simulink library "GNC_math_lib"  (R2022b)
settings: Solver=VariableStepAuto  StartTime=0.0  StopTime=10.0  RelTol=1e-3
settings Model: Creator=David  LastModifiedBy=David

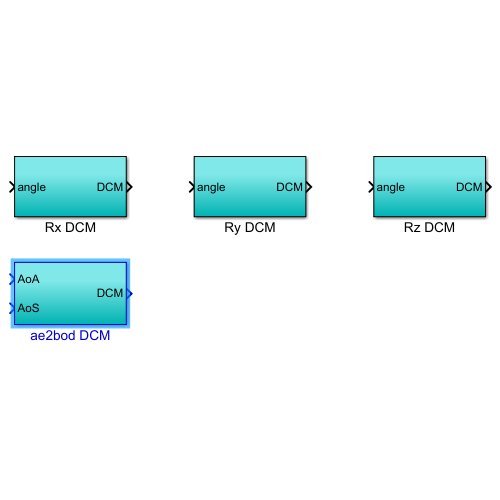
[thumbnail: Simulink's stored preview of the top-level diagram]
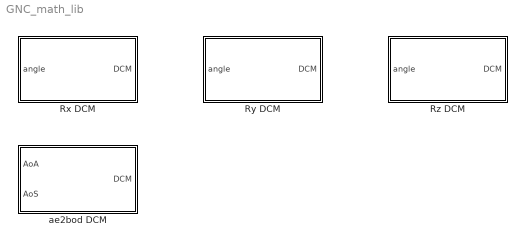
== system GNC_math_lib ==
  Rx DCM : Subsystem
  Ry DCM : Subsystem
  Rz DCM : Subsystem
  ae2bod DCM : Subsystem

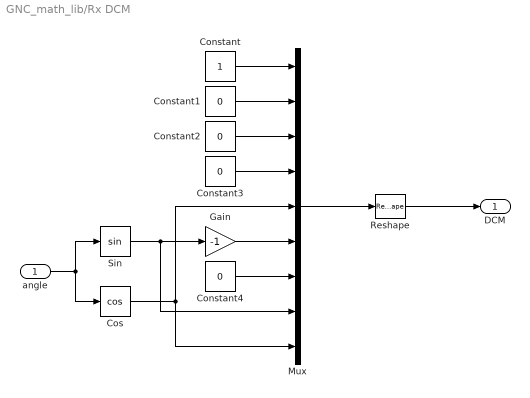
== system GNC_math_lib/Rx DCM ==
  angle : Inport
  Constant : Constant
  Constant{1..4} (4 alike) : Constant  Value=0
  Cos : Trigonometry  Operator=cos
  Gain : Gain  Gain=-1
  Mux : Mux  Inputs=9
  Reshape : Reshape  OutputDimensionality=Customize  OutputDimensions=[3,3]
  Sin : Trigonometry
  DCM : Outport
  wires:
  angle/1 -> Cos/1, Sin/1
  Reshape/1 -> DCM/1
  Mux/1 -> Reshape/1
  Constant/1 -> Mux/1
  Constant1/1 -> Mux/2
  Constant2/1 -> Mux/3
  Constant3/1 -> Mux/4
  Constant4/1 -> Mux/7
  Cos/1 -> Mux/9, Mux/5
  Sin/1 -> Mux/8, Gain/1
  Gain/1 -> Mux/6

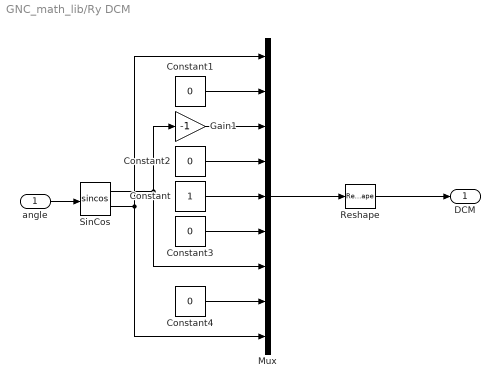
== system GNC_math_lib/Ry DCM ==
  angle : Inport
  Constant : Constant
  Constant{1..4} (4 alike) : Constant  Value=0
  Gain1 : Gain  Gain=-1
  Mux : Mux  Inputs=9
  Reshape : Reshape  OutputDimensionality=Customize  OutputDimensions=[3,3]
  SinCos : Trigonometry  Operator=sincos
  DCM : Outport
  wires:
  angle/1 -> SinCos/1
  Reshape/1 -> DCM/1
  Mux/1 -> Reshape/1
  Constant4/1 -> Mux/8
  Constant3/1 -> Mux/6
  Constant/1 -> Mux/5
  Constant2/1 -> Mux/4
  Constant1/1 -> Mux/2
  SinCos/2 -> Mux/1, Mux/9
  SinCos/1 -> Mux/7, Gain1/1
  Gain1/1 -> Mux/3

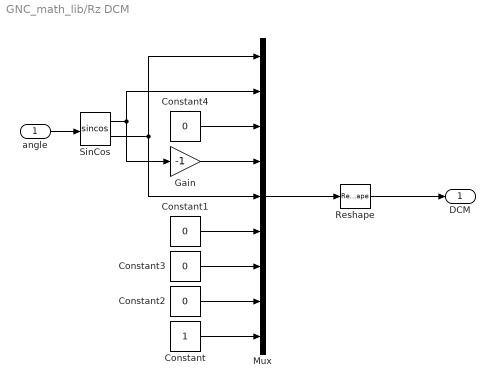
== system GNC_math_lib/Rz DCM ==
  angle : Inport
  Constant : Constant
  Constant{1..4} (4 alike) : Constant  Value=0
  Gain : Gain  Gain=-1
  Mux : Mux  Inputs=9
  Reshape : Reshape  OutputDimensionality=Customize  OutputDimensions=[3,3]
  SinCos : Trigonometry  Operator=sincos
  DCM : Outport
  wires:
  angle/1 -> SinCos/1
  Reshape/1 -> DCM/1
  Mux/1 -> Reshape/1
  Constant/1 -> Mux/9
  Constant3/1 -> Mux/7
  Constant2/1 -> Mux/8
  Constant1/1 -> Mux/6
  Constant4/1 -> Mux/3
  SinCos/1 -> Mux/2, Gain/1
  SinCos/2 -> Mux/5, Mux/1
  Gain/1 -> Mux/4

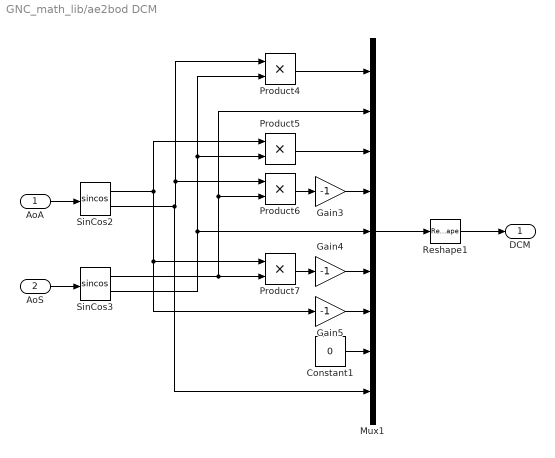
== system GNC_math_lib/ae2bod DCM ==
  AoA : Inport
  AoS : Inport  Port=2
  Constant1 : Constant  Value=0
  Gain3 : Gain  Gain=-1
  Gain4 : Gain  Gain=-1
  Gain5 : Gain  Gain=-1
  Mux1 : Mux  Inputs=9
  Product{4..7} (4 alike) : Product
  Reshape1 : Reshape  OutputDimensionality=Customize  OutputDimensions=[3,3]
  SinCos2 : Trigonometry  Operator=sincos
  SinCos3 : Trigonometry  Operator=sincos
  DCM : Outport
  wires:
  Mux1/1 -> Reshape1/1
  AoS/1 -> SinCos3/1
  AoA/1 -> SinCos2/1
  Reshape1/1 -> DCM/1
  Product4/1 -> Mux1/1
  SinCos2/2 -> Mux1/9, Product6/1, Product4/1
  SinCos3/2 -> Product5/2, Product4/2, Mux1/5
  SinCos3/1 -> Product6/2, Mux1/2, Product7/2
  Product5/1 -> Mux1/3
  SinCos2/1 -> Gain5/1, Product7/1, Product5/1
  Product6/1 -> Gain3/1
  Gain3/1 -> Mux1/4
  Gain4/1 -> Mux1/6
  Product7/1 -> Gain4/1
  Gain5/1 -> Mux1/7
  Constant1/1 -> Mux1/8
